simulink model "feedback_PI"  (R2015b)
settings: Solver=VariableStepAuto  StartTime=0.0  StopTime=0.2  RelTol=1e-3
values from neighbouring files (symbols this model uses):
  A = [0      1       0 ... (first row only)    [top.m]
  B = [0;     0;      1/L]    [top.m]
  C = [1      0       0 ... (first row only)    [top.m]
  D = [0;     0;      0]    [top.m]
settings Model: Creator=Harry  LastModifiedBy=Harry

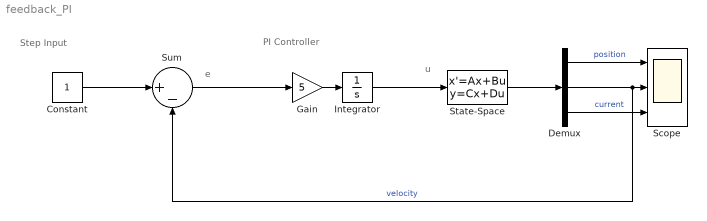
== system feedback_PI ==
  note: e
  note: Step Input
  note: PI Controller
  note: u
  Constant : Constant
  Demux : Demux  Outputs=3
  Gain : Gain  Gain=5
  Integrator : Integrator
  Scope : Scope  NumInputPorts=3
  State-Space : StateSpace  A=A  B=B  C=C  D=D  X0=0
  Sum : Sum  Inputs=|+-
  wires:
  Integrator/1 -> State-Space/1
  Gain/1 -> Integrator/1
  Sum/1 -> Gain/1
  Constant/1 -> Sum/1
  State-Space/1 -> Demux/1
  Demux/2 -> Scope/2, Sum/2  "velocity"
  Demux/3 -> Scope/3  "current"
  Demux/1 -> Scope/1  "position"
